simulink model "LabSystem"  (R2023a)
settings: Solver=ode45  StartTime=0.0  StopTime=1  RelTol=1e-3
values from neighbouring files (symbols this model uses):
  K = 97/5    (= 19.4)    [Parameters.m]
  Kd = (10*sqrt(3)-5)/388    [Parameters.m]
  Kr = 1+0.6/K    (= 1.03092783505)    [Parameters.m]
settings Model: Creator=Jiadong_Hong  LastModifiedBy=Jiadong_Hong

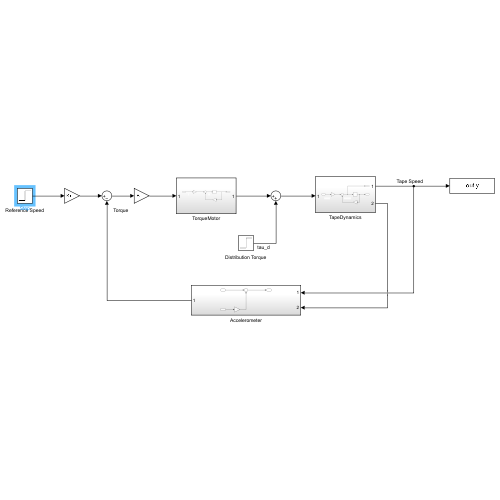
[thumbnail: Simulink's stored preview of the top-level diagram]
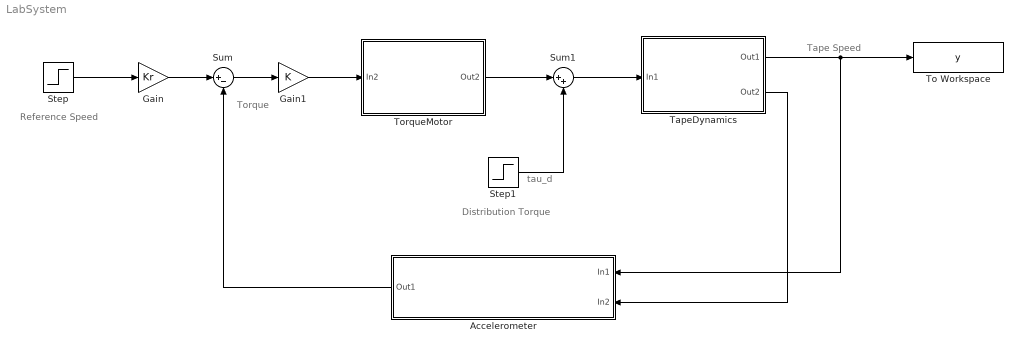
== system LabSystem ==
  note: Torque
  note: tau_d
  note: Reference Speed
  note: Distribution Torque
  note: Tape Speed
  Accelerometer : Subsystem
  Gain : Gain  Gain=Kr
  Gain1 : Gain  Gain=K
  Step : Step  Time=0  After=0  SampleTime=0.01
  Step1 : Step  Time=0  After=0.1  SampleTime=0.01
  Sum : Sum  Inputs=|+-
  Sum1 : Sum  Inputs=|++
  TapeDynamics : Subsystem
  To Workspace : ToWorkspace  VariableName=y  SampleTime=-1
  TorqueMotor : Subsystem
  wires:
  TorqueMotor/1(Out2) -> Sum1/1
  TapeDynamics/1(Out1) -> To Workspace/1, Accelerometer/1(In1)
  Sum1/1 -> TapeDynamics/1(In1)
  Step1/1 -> Sum1/2
  Gain/1 -> Sum/1
  Sum/1 -> Gain1/1
  Step/1 -> Gain/1
  Gain1/1 -> TorqueMotor/1(In2)
  TapeDynamics/2(Out2) -> Accelerometer/2(In2)
  Accelerometer/1(Out1) -> Sum/2

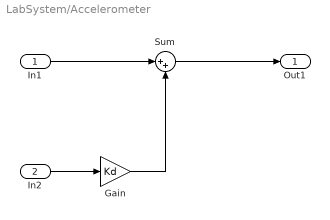
== system LabSystem/Accelerometer ==
  In1 : Inport
  In2 : Inport  Port=2
  Gain : Gain  Gain=Kd
  Sum : Sum  Inputs=|++
  Out1 : Outport
  wires:
  In2/1 -> Gain/1
  Gain/1 -> Sum/2
  In1/1 -> Sum/1
  Sum/1 -> Out1/1

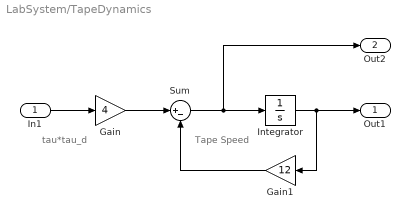
== system LabSystem/TapeDynamics ==
  note: tau*tau_d
  note: Tape Speed
  In1 : Inport
  Gain : Gain  Gain=4
  Gain1 : Gain  Gain=12
  Integrator : Integrator
  Sum : Sum  Inputs=|+-
  Out1 : Outport
  Out2 : Outport  Port=2
  wires:
  Integrator/1 -> Gain1/1, Out1/1
  In1/1 -> Gain/1
  Gain1/1 -> Sum/2
  Gain/1 -> Sum/1
  Sum/1 -> Out2/1, Integrator/1

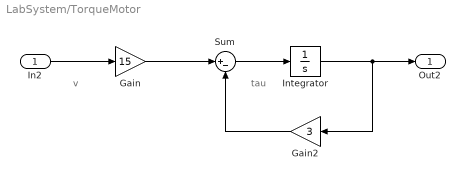
== system LabSystem/TorqueMotor ==
  note: v
  note: tau
  In2 : Inport
  Gain : Gain  Gain=15
  Gain2 : Gain  Gain=3
  Integrator : Integrator
  Sum : Sum  Inputs=|+-
  Out2 : Outport
  wires:
  Integrator/1 -> Out2/1, Gain2/1
  Gain2/1 -> Sum/2
  Sum/1 -> Integrator/1
  In2/1 -> Gain/1
  Gain/1 -> Sum/1
